simulink subsystem "top"  (R2023a)
settings: Solver=VariableStepAuto  StartTime=0.0  StopTime=10.0  RelTol=1e-3
settings Model: Creator=Francesco  LastModifiedBy=Francesco

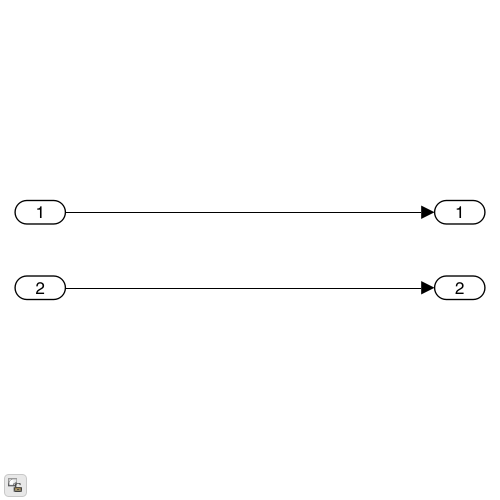
[thumbnail: Simulink's stored preview of the top-level diagram]
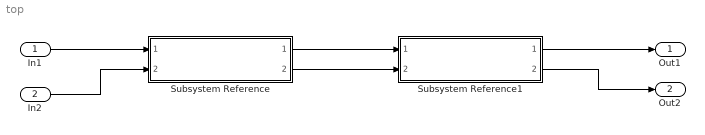
== system top ==
  In1 : Inport
  In2 : Inport  Port=2
  Subsystem Reference : Subsystem  ReferencedSubsystem=modA_ref_sys
  Subsystem Reference1 : Subsystem  ReferencedSubsystem=modB_ref_sys
  Out1 : Outport
  Out2 : Outport  Port=2
  wires:
  In1/1 -> Subsystem Reference/1
  In2/1 -> Subsystem Reference/2
  Subsystem Reference/1 -> Subsystem Reference1/1
  Subsystem Reference/2 -> Subsystem Reference1/2
  Subsystem Reference1/1 -> Out1/1
  Subsystem Reference1/2 -> Out2/1
